simulink model "param_Iden_EKF"  (R2018a)
settings: Solver=ode1  StartTime=0.0  StopTime=20  FixedStep=0.01  RelTol=1e-3
settings Model: Creator=Sarot PC  LastModifiedBy=macuser
settings DataIOCC: ReturnWorkspaceOutputs=on
settings SFSimCC: SimUseLocalCustomCode=on
settings RTWCC: RTWUseLocalCustomCode=on

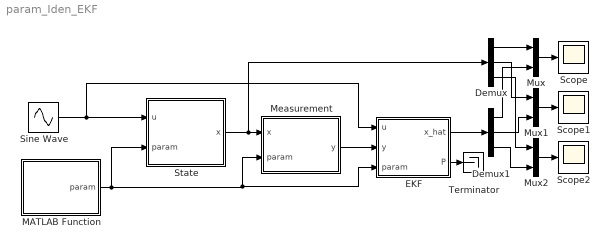
== system param_Iden_EKF ==
  Demux : Demux  Outputs=3
  Demux1 : Demux  Outputs=3
  EKF : MATLAB Function  TreatAsAtomicUnit=on
  MATLAB Function : MATLAB Function  TreatAsAtomicUnit=on
  Measurement : MATLAB Function  TreatAsAtomicUnit=on
  Mux : Mux  Inputs=2
  Mux1 : Mux  Inputs=2
  Mux2 : Mux  Inputs=2
  Scope : Scope
  Scope1 : Scope
  Scope2 : Scope
  Sine Wave : Sin  Frequency=2  SampleTime=0
  State : MATLAB Function  TreatAsAtomicUnit=on
  Terminator : Terminator
  wires:
  MATLAB Function/1(param) -> State/2(param), EKF/3(param), Measurement/2(param)
  State/1(x) -> Demux/1, Measurement/1(x)
  Measurement/1(y) -> EKF/2(y)
  Sine Wave/1 -> EKF/1(u), State/1(u)
  EKF/1(x_hat) -> Demux1/1
  EKF/2(P) -> Terminator/1
  Demux/1 -> Mux/1
  Demux1/1 -> Mux/2
  Demux/2 -> Mux1/1
  Mux/1 -> Scope/1
  Demux1/2 -> Mux1/2
  Demux/3 -> Mux2/1
  Demux1/3 -> Mux2/2
  Mux1/1 -> Scope1/1
  Mux2/1 -> Scope2/1

== matlab function param_Iden_EKF/State ==
  settings: updateMethod=DISCRETE
  data: u input; x output; param input
function x = fcn(u,param)

persistent x_
if isempty(x_),x_ = [0;10;100];end
n = param(1);
dt = param(2);
Q = reshape(param(3:2+n*n),n,n);

x = x_ + [-x_(1)*x_(2)+x_(3)*u;0;0]*dt+sqrt(dt)*sqrt(Q)*randn(n,1);
x_= x;

== matlab function param_Iden_EKF/MATLAB Function ==
  data: param output
function param = fcn

n  = 3;
m  = 1;
dt = 0.01;

Q = 1e-6*diag([1 10 100]);
R = 1e-3;

param = [n;dt;reshape(Q,[],1);m;reshape(R,[],1)];

== matlab function param_Iden_EKF/Measurement ==
  data: x input; y output; param input
function y = fcn(x,param)

n = param(1);
m = 1;%param(4+n*n);
R = reshape(param(4+n*n:3+n*n+m*m),m,m);

C = [1 0 0];

y = C*x+sqrt(R)*randn(m,1);

== matlab function param_Iden_EKF/EKF ==
  settings: updateMethod=DISCRETE
  data: u input; x_hat output; P output; y input; param input
function [x_hat,P] = fcn(u,y,param)

n = param(1);
dt = param(2);
Q = reshape(param(3:2+n*n),n,n);
m = param(3+n*n);
R = reshape(param(4+n*n:3+n*n+m*m),m,m);

persistent x_ P_
if isempty(x_), x_= randn(n,1); P_ = 1e-1*eye(n);end

A = [1-x_(2)*dt -x_(1)*dt u*dt; 0 1 0; 0 0 1];
C = [1 0 0];

x = x_ + [-x_(1)*x_(2)+x_(3)*u;0;0]*dt; 
x_hat = x;
P = A*P_*A'+Q+1e-5*diag([1 1000 10000]);

W = (P*C')/(C*P*C'+10*R);
x_ = x + W*(y-C*x);
P_ = P - W*C*P;
